simulink model "SimplePipeMessagesMDL"  (R2013a)
settings: Solver=ode45  StartTime=0.0  StopTime=1800  RelTol=1e-3
undefined symbols (not defined in the file or in its folder): CarnotCallbacks_SimplePipeMessages
libraries: carnot x1
settings Model: Creator=awohlfei  LastModifiedBy=awohlfei

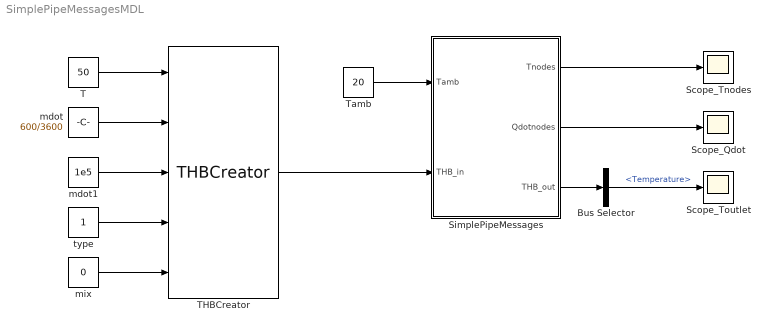
== system SimplePipeMessagesMDL ==
  Bus Selector : BusSelector  OutputSignals=Temperature
  Scope_Qdot : Scope
  Scope_Tnodes : Scope
  Scope_Toutlet : Scope
      settings: TimeRange=1800  SaveName=ScopeData2
  SimplePipeMessages : Subsystem  LoadFcn=CarnotCallbacks_SimplePipeMessages('LoadFcn', gcb);  mask{UA=100, VOLUME=0.1, TINIT=[20 25 30 35 40], NODES=5, MESSAGELEVELBLOCK=DEBUGLEVEL, MAXTOTALMESSAGES=inf, MAXCONSECUTIVEMESSAGES=inf, WRITETOFILE=0, MESSAGEFILENAME='bla.txt'}
      mask prompts: UA "heat transfer coefficient [W/K]"; VOLUME "volume of pipe [m³]"; TINIT "initial temperature [°C]"; NODES "number of nodes [1]"; MESSAGELEVELBLOCK "message level of block"; MAXTOTALMESSAGES "maximum number of messages"; MAXCONSECUTIVEMESSAGES "number of consecutive messages"; WRITETOFILE "write messages to file"; MESSAGEFILENAME "filename for messages"
      mask init:
      | if UA<0.0
      |     error('UA must be >=0 W/K !');
      | end
      | 
      | if VOLUME<0.0
      |     error('Volume must be >= 0 m³ !');
      | end
      | 
      | if (double(int32(NODES))-NODES)>eps(NODES)
      |     error('The number of nodes must be an integer!');
      | end
      | 
      | if NODES < 1
      |     error('The number of nodes must be positive!');
      | end
      | 
      | if sum(TINIT<-273.15)>0
      |     error('Initial temperature must be >= -273.15 °C !');
      | end
      | 
      | if numel(TINIT)~=NODES
      |     if numel(TINIT) == 1
      |         TINIT = ones(NODES, 1)*TINIT;
      |     else
      |         error('The initial temperature must have number of nodes elements or one!');
      |     end
      | end
      | 
      | 
      | %check for global message settings
      | [MESSAGELEVELBLOCK, MAXTOTALMESSAGES, MAXCONSECUTIVEMESSAGES, WRITETOFILE, MESSAGEFILENAME] = CarnotCallbacks_SimplePipeMessages('CheckDebugLevels', MESSAGELEVELBLOCK, MAXTOTALMESSAGES, MAXCONSECUTIVEMESSAGES, WRITETOFILE, MESSAGEFILENAME);
      mask Callback UA:
      | %set the visibility of the message parameters
      | CarnotCallbacks_SimplePipeMessages('MaskVisibilities', gcb);
      mask TypeOptions MESSAGELEVELBLOCK: DEBUGLEVEL | INFOLEVEL | WARNINGLEVEL | ERRORLEVEL | FATALLEVEL | NOLEVEL | HALLO
  T : Constant  Value=50
  THBCreator : carnot/Basic/Hydraulics/THBCreator  Inport_ID=off  Inport_T=on  Inport_mdot=on  Inport_p=on  Inport_type=on  Inport_mix=on  Inport_d=off  Inport_c=off  Inport_l=off  Inport_q=off  Inport_LH=off  Inport_H=off  ID=20001  T=20  mdot=0  p=1e5  FluidType=1  FluidMix=0  d=0.01  c=0  l=0  q=0  LH=0  H=0  Annotation_ID=off  Annotation_T=off  Annotation_mdot=off  Annotation_p=off  Annotation_type=off  Annotation_mix=off  Annotation_d=off  Annotation_c=off  Annotation_l=off  Annotation_q=off  Annotation_LH=off  Annotation_H=off
  Tamb : Constant  Value=20
  mdot : Constant  Value=600/3600
  mdot1 : Constant  Value=1e5
  mix : Constant  Value=0
  type : Constant
  wires:
  T/1 -> THBCreator/1
  mdot/1 -> THBCreator/2
  mdot1/1 -> THBCreator/3
  type/1 -> THBCreator/4
  mix/1 -> THBCreator/5
  THBCreator/1 -> SimplePipeMessages/2(THB_in)
  Tamb/1 -> SimplePipeMessages/1(Tamb)
  SimplePipeMessages/3(THB_out) -> Bus Selector/1
  SimplePipeMessages/1(Tnodes) -> Scope_Tnodes/1
  SimplePipeMessages/2(Qdotnodes) -> Scope_Qdot/1
  Bus Selector/1 -> Scope_Toutlet/1  "<Temperature>"

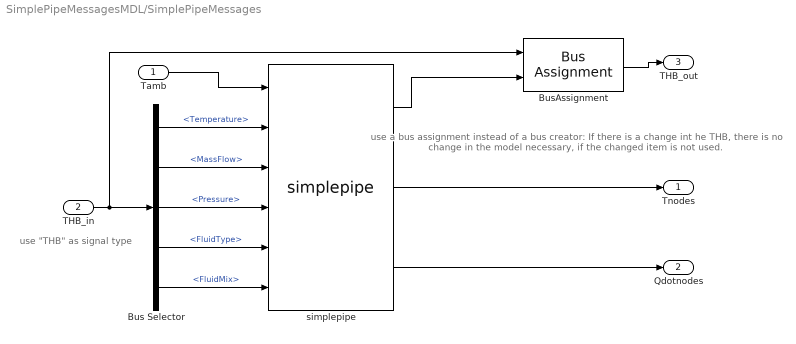
== system SimplePipeMessagesMDL/SimplePipeMessages ==
  note: use a bus assignment instead of a bus creator:
      | If there is a change int he THB,
      | there is no change in the model necessary, if
      | the changed item is not used.
  note: use "THB" as signal type
  Tamb : Inport
  THB_in : Inport  Port=2  OutDataTypeStr=Bus: THB
  Bus Selector : BusSelector  OutputSignals=Temperature,MassFlow,Pressure,FluidType,FluidMix
  BusAssignment : BusAssignment  AssignedSignals=Temperature
  simplepipe : S-Function  FunctionName=simplepipe  Parameters=UA, VOLUME, NODES, TINIT  EnableBusSupport=off
  Tnodes : Outport
  Qdotnodes : Outport  Port=2
  THB_out : Outport  Port=3
  wires:
  THB_in/1 -> BusAssignment/1, Bus Selector/1
  Tamb/1 -> simplepipe/1
  Bus Selector/1 -> simplepipe/2  "<Temperature>"
  Bus Selector/2 -> simplepipe/3  "<MassFlow>"
  Bus Selector/3 -> simplepipe/4  "<Pressure>"
  Bus Selector/4 -> simplepipe/5  "<FluidType>"
  Bus Selector/5 -> simplepipe/6  "<FluidMix>"
  BusAssignment/1 -> THB_out/1
  simplepipe/1 -> BusAssignment/2
  simplepipe/2 -> Tnodes/1
  simplepipe/3 -> Qdotnodes/1
